simulink library "Memory_Blocks_Lib"  (Simulink 8.7)
settings: Solver=ode45  StartTime=0.0  StopTime=10.0  RelTol=1e-3
libraries: Memory_Blocks_Lib x72, simulink_extras x26, Decoders_Lib x7, Bit_Multiplexers_Lib x5, Byte_Multiplexers_Lib x2, Word_Multiplexers_Lib x1, commutil2 x1
(part 2 of 2)

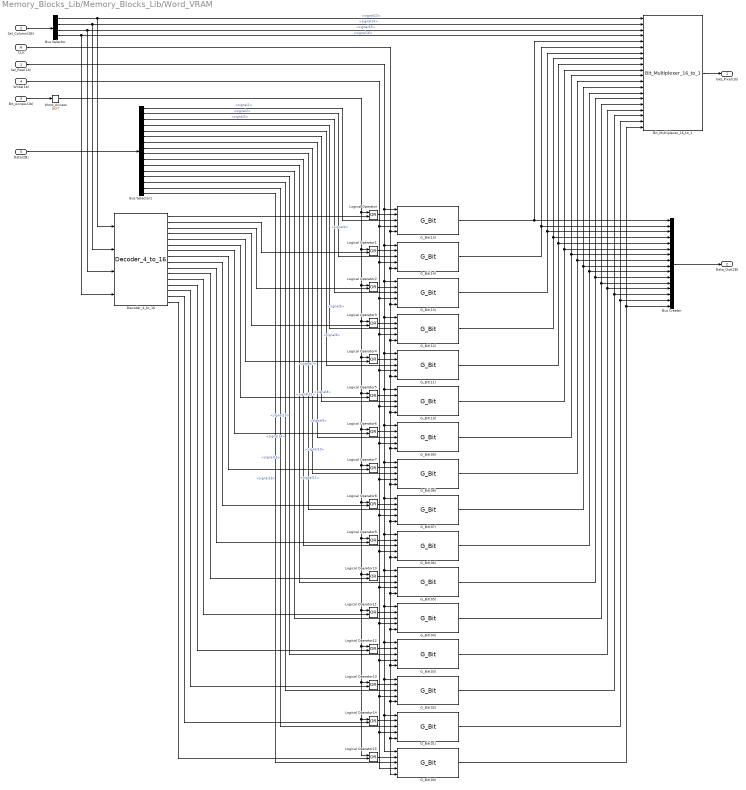
== system Memory_Blocks_Lib/Memory_Blocks_Lib/Word_VRAM ==
  Sel_Raw(1b) : Inport
  Sel_Column(2B) : Inport  Port=2
  Bit_Access(1b) : Inport  Port=3
  Write(1b) : Inport  Port=4
  Data(2B) : Inport  Port=5
  CLK : Inport  Port=6
  Bit_Multiplexer_16_to_1 : Bit_Multiplexers_Lib/Bit_Multiplexers_Lib/Bit_Multiplexer_16_to_1
  Bus Creator : BusCreator  Inputs=16
  Bus Selector : BusSelector  OutputSignals=signal13,signal14,signal15,signal16
  Bus Selector1 : BusSelector  OutputSignals=signal1,signal2,signal3,signal4,signal5,signal6,signal7,signal8,signal9,signal10,signal11,signal12,signal13,signal14,signal15,signal16
  Decoder_4_to_16 : Decoders_Lib/Decoders_Lib/Decoder_4_to_16
  G_Bit(00) : Memory_Blocks_Lib/Memory_Blocks_Lib/G_Bit
  G_Bit(01) : Memory_Blocks_Lib/Memory_Blocks_Lib/G_Bit
  G_Bit(02) : Memory_Blocks_Lib/Memory_Blocks_Lib/G_Bit
  G_Bit(03) : Memory_Blocks_Lib/Memory_Blocks_Lib/G_Bit
  G_Bit(04) : Memory_Blocks_Lib/Memory_Blocks_Lib/G_Bit
  G_Bit(05) : Memory_Blocks_Lib/Memory_Blocks_Lib/G_Bit
  G_Bit(06) : Memory_Blocks_Lib/Memory_Blocks_Lib/G_Bit
  G_Bit(07) : Memory_Blocks_Lib/Memory_Blocks_Lib/G_Bit
  G_Bit(08) : Memory_Blocks_Lib/Memory_Blocks_Lib/G_Bit
  G_Bit(09) : Memory_Blocks_Lib/Memory_Blocks_Lib/G_Bit
  G_Bit(10) : Memory_Blocks_Lib/Memory_Blocks_Lib/G_Bit
  G_Bit(11) : Memory_Blocks_Lib/Memory_Blocks_Lib/G_Bit
  G_Bit(12) : Memory_Blocks_Lib/Memory_Blocks_Lib/G_Bit
  G_Bit(13) : Memory_Blocks_Lib/Memory_Blocks_Lib/G_Bit
  G_Bit(14) : Memory_Blocks_Lib/Memory_Blocks_Lib/G_Bit
  G_Bit(15) : Memory_Blocks_Lib/Memory_Blocks_Lib/G_Bit
  Logical Operator{,1..15} (16 alike) : Logic  Operator=OR  IconShape=distinctive  AllPortsSameDT=off  OutDataTypeStr=boolean
  Word_Access : Logic  Operator=NOT  IconShape=distinctive  AllPortsSameDT=off  OutDataTypeStr=boolean
  Get_Pixel(1b) : Outport
  Data_Out(2B) : Outport  Port=2
  wires:
  Bit_Access(1b)/1 -> Word_Access/1
  Word_Access/1 -> Logical Operator/1, Logical Operator15/1, Logical Operator14/1, Logical Operator13/1, Logical Operator12/1, Logical Operator11/1, Logical Operator10/1, Logical Operator9/1, Logical Operator8/1, Logical Operator7/1, Logical Operator6/1, Logical Operator5/1, Logical Operator4/1, Logical Operator3/1, Logical Operator2/1, Logical Operator1/1
  Logical Operator15/1 -> G_Bit(00)/2
  Logical Operator14/1 -> G_Bit(01)/2
  Logical Operator13/1 -> G_Bit(02)/2
  Logical Operator12/1 -> G_Bit(03)/2
  Logical Operator11/1 -> G_Bit(04)/2
  Logical Operator10/1 -> G_Bit(05)/2
  Logical Operator9/1 -> G_Bit(06)/2
  Logical Operator8/1 -> G_Bit(07)/2
  Logical Operator7/1 -> G_Bit(08)/2
  Logical Operator6/1 -> G_Bit(09)/2
  Logical Operator5/1 -> G_Bit(10)/2
  Logical Operator4/1 -> G_Bit(11)/2
  Logical Operator3/1 -> G_Bit(12)/2
  Logical Operator2/1 -> G_Bit(13)/2
  Logical Operator1/1 -> G_Bit(14)/2
  Logical Operator/1 -> G_Bit(15)/2
  Bit_Multiplexer_16_to_1/1 -> Get_Pixel(1b)/1
  Write(1b)/1 -> G_Bit(15)/4, G_Bit(14)/4, G_Bit(13)/4, G_Bit(12)/4, G_Bit(11)/4, G_Bit(10)/4, G_Bit(09)/4, G_Bit(08)/4, G_Bit(07)/4, G_Bit(06)/4, G_Bit(05)/4, G_Bit(04)/4, G_Bit(03)/4, G_Bit(02)/4, G_Bit(01)/4, G_Bit(00)/4
  Bus Creator/1 -> Data_Out(2B)/1
  G_Bit(00)/1 -> Bus Creator/16, Bit_Multiplexer_16_to_1/20
  G_Bit(01)/1 -> Bus Creator/15, Bit_Multiplexer_16_to_1/19
  G_Bit(02)/1 -> Bus Creator/14, Bit_Multiplexer_16_to_1/18
  G_Bit(03)/1 -> Bus Creator/13, Bit_Multiplexer_16_to_1/17
  G_Bit(04)/1 -> Bus Creator/12, Bit_Multiplexer_16_to_1/16
  G_Bit(05)/1 -> Bus Creator/11, Bit_Multiplexer_16_to_1/15
  G_Bit(06)/1 -> Bus Creator/10, Bit_Multiplexer_16_to_1/14
  G_Bit(07)/1 -> Bus Creator/9, Bit_Multiplexer_16_to_1/13
  G_Bit(08)/1 -> Bus Creator/8, Bit_Multiplexer_16_to_1/12
  G_Bit(09)/1 -> Bus Creator/7, Bit_Multiplexer_16_to_1/11
  G_Bit(10)/1 -> Bus Creator/6, Bit_Multiplexer_16_to_1/10
  G_Bit(11)/1 -> Bus Creator/5, Bit_Multiplexer_16_to_1/9
  G_Bit(12)/1 -> Bus Creator/4, Bit_Multiplexer_16_to_1/8
  G_Bit(13)/1 -> Bus Creator/3, Bit_Multiplexer_16_to_1/7
  G_Bit(14)/1 -> Bus Creator/2, Bit_Multiplexer_16_to_1/6
  G_Bit(15)/1 -> Bus Creator/1, Bit_Multiplexer_16_to_1/5
  Sel_Raw(1b)/1 -> G_Bit(15)/1, G_Bit(14)/1, G_Bit(13)/1, G_Bit(12)/1, G_Bit(11)/1, G_Bit(10)/1, G_Bit(09)/1, G_Bit(08)/1, G_Bit(07)/1, G_Bit(06)/1, G_Bit(05)/1, G_Bit(04)/1, G_Bit(03)/1, G_Bit(02)/1, G_Bit(00)/1, G_Bit(01)/1
  Bus Selector/4 -> Bit_Multiplexer_16_to_1/4, Decoder_4_to_16/4  "<signal16>"
  Bus Selector/2 -> Bit_Multiplexer_16_to_1/2, Decoder_4_to_16/2  "<signal14>"
  Decoder_4_to_16/14 -> Logical Operator13/2
  Decoder_4_to_16/12 -> Logical Operator11/2
  Decoder_4_to_16/10 -> Logical Operator9/2
  Decoder_4_to_16/15 -> Logical Operator14/2
  Decoder_4_to_16/13 -> Logical Operator12/2
  Decoder_4_to_16/16 -> Logical Operator15/2
  Decoder_4_to_16/9 -> Logical Operator8/2
  Decoder_4_to_16/5 -> Logical Operator4/2
  Decoder_4_to_16/7 -> Logical Operator6/2
  Decoder_4_to_16/4 -> Logical Operator3/2
  Decoder_4_to_16/11 -> Logical Operator10/2
  Decoder_4_to_16/3 -> Logical Operator2/2
  Bus Selector/3 -> Bit_Multiplexer_16_to_1/3, Decoder_4_to_16/3  "<signal15>"
  CLK/1 -> G_Bit(15)/5, G_Bit(14)/5, G_Bit(13)/5, G_Bit(12)/5, G_Bit(11)/5, G_Bit(10)/5, G_Bit(09)/5, G_Bit(08)/5, G_Bit(07)/5, G_Bit(06)/5, G_Bit(05)/5, G_Bit(04)/5, G_Bit(03)/5, G_Bit(02)/5, G_Bit(01)/5, G_Bit(00)/5
  Sel_Column(2B)/1 -> Bus Selector/1
  Decoder_4_to_16/1 -> Logical Operator/2
  Decoder_4_to_16/2 -> Logical Operator1/2
  Decoder_4_to_16/6 -> Logical Operator5/2
  Decoder_4_to_16/8 -> Logical Operator7/2
  Bus Selector/1 -> Decoder_4_to_16/1, Bit_Multiplexer_16_to_1/1  "<signal13>"
  Data(2B)/1 -> Bus Selector1/1
  Bus Selector1/16 -> G_Bit(00)/3  "<signal16>"
  Bus Selector1/15 -> G_Bit(01)/3  "<signal15>"
  Bus Selector1/14 -> G_Bit(02)/3  "<signal14>"
  Bus Selector1/13 -> G_Bit(03)/3  "<signal13>"
  Bus Selector1/12 -> G_Bit(04)/3  "<signal12>"
  Bus Selector1/11 -> G_Bit(05)/3  "<signal11>"
  Bus Selector1/10 -> G_Bit(06)/3  "<signal10>"
  Bus Selector1/9 -> G_Bit(07)/3  "<signal9>"
  Bus Selector1/8 -> G_Bit(08)/3  "<signal8>"
  Bus Selector1/7 -> G_Bit(09)/3  "<signal7>"
  Bus Selector1/6 -> G_Bit(10)/3  "<signal6>"
  Bus Selector1/5 -> G_Bit(11)/3  "<signal5>"
  Bus Selector1/4 -> G_Bit(12)/3  "<signal4>"
  Bus Selector1/3 -> G_Bit(13)/3  "<signal3>"
  Bus Selector1/2 -> G_Bit(14)/3  "<signal2>"
  Bus Selector1/1 -> G_Bit(15)/3  "<signal1>"
